simulink model "Par11_2_4_20210318S"  (R2018a)
settings: Solver=VariableStepAuto  StartTime=0.0  StopTime=10.0  RelTol=1e-3
settings Model: Creator=wangluo  LastModifiedBy=wangluo

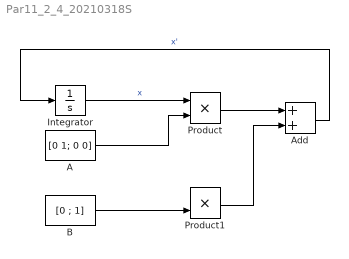
== system Par11_2_4_20210318S ==
  A : Constant  Value=[0 1; 0 0]
  Add : Sum
  B : Constant  Value=[0 ; 1]
  Integrator : Integrator
  Product : Product
  Product1 : Product
  wires:
  A/1 -> Product/2
  Integrator/1 -> Product/1  "x"
  Product/1 -> Add/1
  Product1/1 -> Add/2
  Add/1 -> Integrator/1  "x'"
  B/1 -> Product1/2
